simulink model "FIVE_LEVEL_INV"  (R2015a)
settings: Solver=ode3  StartTime=0.0  StopTime=10.0  RelTol=1e-3
libraries: powerlib x13, arduinolib x8
settings Model: ExtModeTrigDuration=2  Creator=Anand  LastModifiedBy=AKGC
settings OptimizationCC: OptimizeModelRefInitCode=on  LifeSpan=1
settings DebuggingCC: UnderspecifiedInitializationDetection=Classic  MergeDetectMultiDrivingBlocksExec=none
settings HardwareCC: ProdBitPerInt=16  ProdBitPerPointer=8  ProdIntDivRoundTo=Zero  ProdEndianess=LittleEndian  ProdWordSize=8  ProdHWDeviceType=Atmel->AVR
settings RTWCC: SystemTargetFile=realtime.tlc  GenerateMakefile=off  TemplateMakefile=realtime.tmf  Description=Run on Target Hardware  RTWVerbose=off
settings ERTTargetCC: CombineOutputUpdateFcns=off  ExtModeTransport=3  ExtModeMexFile=ext_serial_win32_comm_rtt  ExtModeMexArgs=0 1 9600  ERTSrcFileBannerTemplate=realtime_code_template.cgt  ERTHdrFileBannerTemplate=realtime_code_template.cgt  ERTDataSrcFileTemplate=realtime_code_template.cgt  ERTDataHdrFileTemplate=realtime_code_template.cgt  ERTCustomFileTemplate=realtime_file_process.tlc

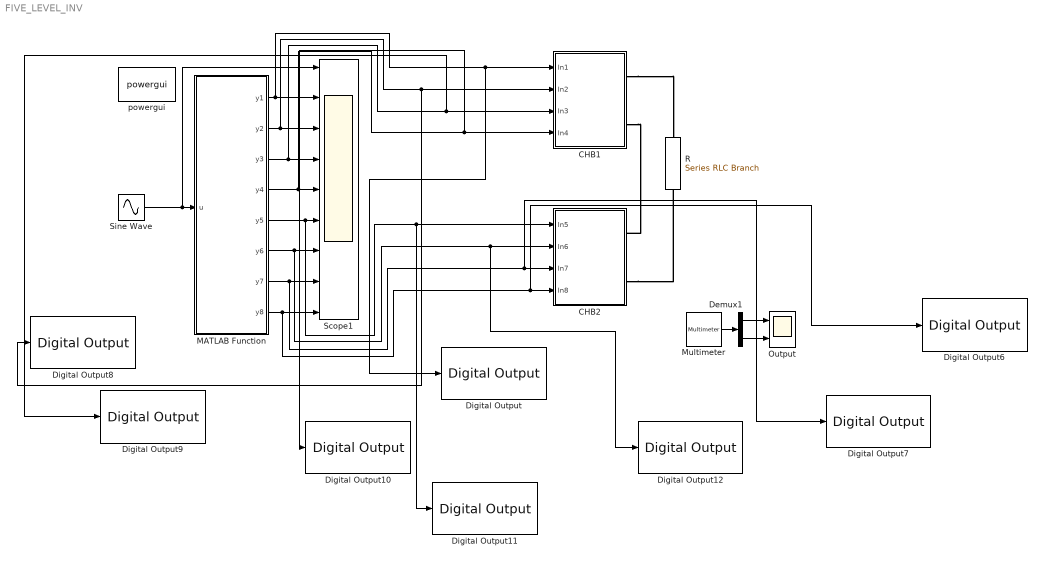
== system FIVE_LEVEL_INV ==
  CHB1 : Subsystem
  CHB2 : Subsystem
  Demux1 : Demux  Outputs=2
  Digital Output : arduinolib/Digital Output  pinNumber=22  blockPlatform=arduino
  Digital Output10 : arduinolib/Digital Output  pinNumber=25  blockPlatform=arduino
  Digital Output11 : arduinolib/Digital Output  pinNumber=26  blockPlatform=arduino
  Digital Output12 : arduinolib/Digital Output  pinNumber=27  blockPlatform=arduino
  Digital Output6 : arduinolib/Digital Output  pinNumber=29  blockPlatform=arduino
  Digital Output7 : arduinolib/Digital Output  pinNumber=28  blockPlatform=arduino
  Digital Output8 : arduinolib/Digital Output  pinNumber=23  blockPlatform=arduino
  Digital Output9 : arduinolib/Digital Output  pinNumber=24  blockPlatform=arduino
  MATLAB Function : MATLAB Function  TreatAsAtomicUnit=on
  Multimeter : powerlib/Measurements/Multimeter  PhasorSimulation=off  OutputType=Complex  sel=[1 2]  L=2  Gain=[1 1]  yselected={'Ub: R','Ib: R'};  PSBOutputType=1  PSBequivalent=0  AxesSetting=[0,0.1,-100,100]  Display=0  SavedBlockNames=-11
  Output : Scope  NumInputPorts=2
      settings: YMin=-5~-5  YMax=5~5  SaveName=ScopeData2
  R : powerlib/Elements/Series RLC Branch  LConnTagsString=__new0  RConnTagsString=__new0  BranchType=R  Resistance=1  Inductance=1e-3  SetiL0=off  InitialCurrent=0  Capacitance=1e-6  Setx0=off  InitialVoltage=0  Measurements=Branch voltage and current
  Scope1 : Scope  NumInputPorts=9
      settings: YMin=-5~-5~-5~-5~-5~-5~-5~-5~-5  YMax=5~5~5~5~5~5~5~5~5
  Sine Wave : Sin  Amplitude=5  Frequency=314.159265  SampleTime=0.000555
  powergui : powerlib/powergui  Priority=1  SimulationMode=Continuous  SolverType=Tustin/Backward Euler (TBE)  SampleTime=50e-6  frequency=60  SPID=off  DisableSnubberDevices=off  DisableRonSwitches=off  DisableVfSwitches=off  SwTol=0  DisplayEquations=off  Interpol=off  methode=off  Ts=100  FunctionMessages=off  echomessages=off  HookPort=off  EnableUseOfTLC=off  x0status=blocks  frequencyindice=0  Pbase=100e6  ErrMax=1e-4  Iterations=50  UnitsV=kV  UnitsW=MW  buscounter=0  RestoreLinks=warning  ResistiveCurrentMeasurement=off  Frange=[0:2:500]  Ylog=off  Xlog=on  ShowGrid=off  save=off  variable=ZData  structure=0  ZoomFFT=off  StartTime=0.0  cycles=1  DisplayStyle=1  fundamental=60  FreqAxis=off  MaxFrequency=1000  frequencyindicesteady=1  RmsSteady=1  display=off
  wires:
  Sine Wave/1 -> MATLAB Function/1(u), Scope1/1
  MATLAB Function/1(y1) -> Digital Output/1, CHB1/1(In1), Scope1/2
  MATLAB Function/4(y4) -> Digital Output10/1, CHB1/4(In4), Scope1/5
  MATLAB Function/5(y5) -> CHB2/1(In5), Digital Output11/1, Scope1/6
  MATLAB Function/6(y6) -> Digital Output12/1, CHB2/2(In6), Scope1/7
  MATLAB Function/7(y7) -> Digital Output7/1, CHB2/3(In7), Scope1/8
  MATLAB Function/8(y8) -> Digital Output6/1, CHB2/4(In8), Scope1/9
  Demux1/1 -> Output/1
  Demux1/2 -> Output/2
  Multimeter/1 -> Demux1/1
  MATLAB Function/2(y2) -> Digital Output8/1, CHB1/2(In2), Scope1/3
  MATLAB Function/3(y3) -> Digital Output9/1, CHB1/3(In3), Scope1/4
  connections:
  CHB1/RConn2 -- CHB2/RConn1
  CHB1/RConn1 -- R/LConn1
  CHB2/RConn2 -- R/RConn1

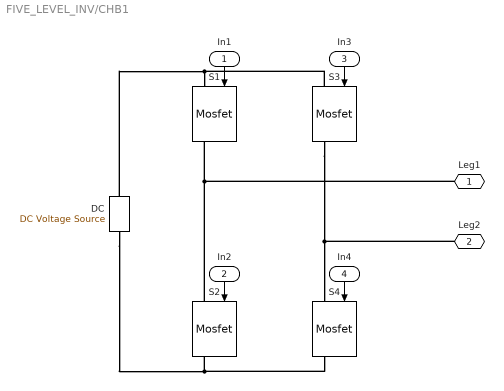
== system FIVE_LEVEL_INV/CHB1 ==
  In1 : Inport
  In2 : Inport  Port=2
  In3 : Inport  Port=3
  In4 : Inport  Port=4
  "DC " : powerlib/Electrical Sources/DC Voltage Source  Amplitude=100  Measurements=None
  S{1..4} (4 alike) : powerlib/Power Electronics/Mosfet  Ron=0.1  Lon=0  Rd=0.01  Vfd=0  IC=0  Rs=1e5  Cs=inf  Measurements=on
  Leg1 : PMIOPort  Port=1  Side=Right
  Leg2 : PMIOPort  Port=2  Side=Right
  wires:
  In2/1 -> S2/1
  In3/1 -> S3/1
  In4/1 -> S4/1
  In1/1 -> S1/1
  connections:
  S2/RConn1 -- S4/RConn1 -- "DC "/LConn1
  S2/LConn1 -- S1/RConn1 -- Leg1/RConn1
  S3/RConn1 -- Leg2/RConn1 -- S4/LConn1
  S1/LConn1 -- "DC "/RConn1 -- S3/LConn1

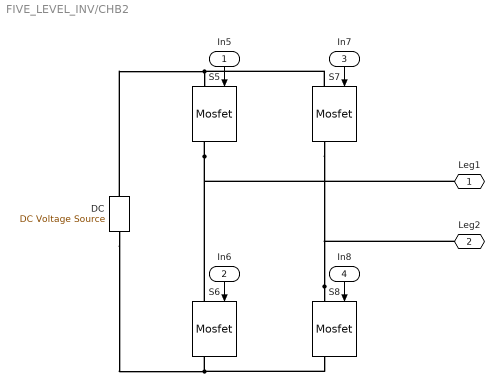
== system FIVE_LEVEL_INV/CHB2 ==
  In5 : Inport
  In6 : Inport  Port=2
  In7 : Inport  Port=3
  In8 : Inport  Port=4
  "DC " : powerlib/Electrical Sources/DC Voltage Source  Amplitude=100  Measurements=None
  S{5..8} (4 alike) : powerlib/Power Electronics/Mosfet  Ron=0.1  Lon=0  Rd=0.01  Vfd=0  IC=0  Rs=1e5  Cs=inf  Measurements=on
  Leg1 : PMIOPort  Port=1  Side=Right
  Leg2 : PMIOPort  Port=2  Side=Right
  wires:
  In5/1 -> S5/1
  In8/1 -> S8/1
  In7/1 -> S7/1
  In6/1 -> S6/1
  connections:
  "DC "/RConn1 -- S5/LConn1 -- S7/LConn1
  S8/LConn1 -- Leg2/RConn1 -- S7/RConn1
  S5/RConn1 -- Leg1/RConn1 -- S6/LConn1
  S8/RConn1 -- S6/RConn1 -- "DC "/LConn1

== matlab function FIVE_LEVEL_INV/MATLAB Function ==
  data: u input; y1 output; y2 output; y3 output; y4 output; y5 output; y6 output; y7 output; y8 output
function [y1,y2,y3,y4,y5,y6,y7,y8] = fcn(u)

%Positive Cycle
        if(u>=0 && u<=1)
            y1=0; y2=0;y3=0; y4=0;y5=0;y6=0;y7=0;y8=0;      %Vo=0
        elseif(u>=1 && u<=3)
            y1=1; y2=0;y3=0; y4=1;y5=0;y6=1;y7=0;y8=1;      %Vo=+V1
        elseif(u>=3 && u<=7)
            y1=1; y2=0;y3=0; y4=1;y5=1;y6=0;y7=0;y8=1;      %Vo=+(V1+V2)
        elseif(u>=7 && u<=9)
            y1=1; y2=0;y3=0; y4=1;y5=0;y6=1;y7=0;y8=1;      %Vo=+V1
        elseif(u>=9 && u<=10)
            y1=0; y2=0;y3=0; y4=0;y5=0;y6=0;y7=0;y8=0;      %Vo=0
 %Negative Cycle
        elseif(u<=-0 && u>=-1)
            y1=0; y2=0;y3=0; y4=0;y5=0;y6=0;y7=0;y8=0;    %Vo=0
        elseif(u<=-1 && u>=-3)
            y1=0; y2=1;y3=1; y4=0;y5=1;y6=0;y7=1;y8=0;     %Vo=+V1
        elseif(u<=-3 && u>=-7)
            y1=0; y2=1;y3=1; y4=0;y5=0;y6=1;y7=1;y8=0;     %Vo=+(V1+V2)
        elseif(u<=-9 && u>=-10)
            y1=0; y2=1;y3=1; y4=0;y5=1;y6=0;y7=1;y8=0;    %Vo=0
        else
           y1=0; y2=0;y3=0; y4=0;y5=0;y6=0;y7=0;y8=0;   %Vo=0
        end
